simulink model "Neurofeedback_ErrorFunction"  (R2021b)
settings: Solver=VariableStepAuto  StartTime=0.0  StopTime=30  RelTol=1e-3
settings Model: Creator=mariodelossantos  LastModifiedBy=mariodelossantos

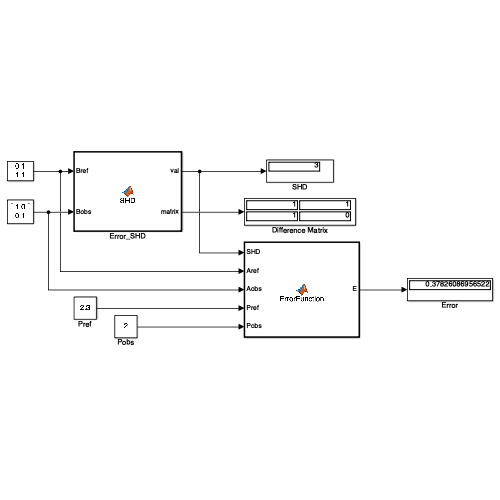
[thumbnail: Simulink's stored preview of the top-level diagram]
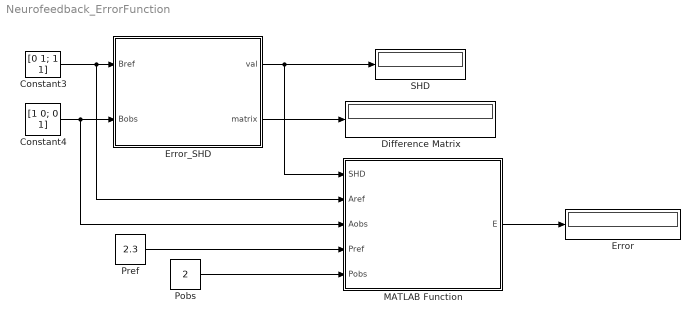
== system Neurofeedback_ErrorFunction ==
  Constant3 : Constant  Value=[0 1; 1 1]
  Constant4 : Constant  Value=[1 0; 0 1]
  Difference Matrix : Display
  Error : Display
  Error_SHD : MATLAB Function  TreatAsAtomicUnit=on
  MATLAB Function : MATLAB Function  TreatAsAtomicUnit=on
  Pobs : Constant  Value=2
  Pref : Constant  Value=2.3
  SHD : Display
  wires:
  Constant4/1 -> MATLAB Function/3(Aobs), Error_SHD/2(Bobs)
  Error_SHD/1(val) -> MATLAB Function/1(SHD), SHD/1
  Error_SHD/2(matrix) -> Difference Matrix/1
  Constant3/1 -> MATLAB Function/2(Aref), Error_SHD/1(Bref)
  MATLAB Function/1(E) -> Error/1
  Pref/1 -> MATLAB Function/4(Pref)
  Pobs/1 -> MATLAB Function/5(Pobs)

== matlab function Neurofeedback_ErrorFunction/Error_SHD ==
  data: Bref input; val output; Bobs input; matrix output
function [val,matrix]=SHD(Bref,Bobs)

val = sum(sum(xor(Bref,Bobs)));
matrix = xor(Bref,Bobs);

== matlab function Neurofeedback_ErrorFunction/MATLAB Function ==
  data: SHD input; Aref input; E output; Aobs input; Pref input; Pobs input
function E  = ErrorFunction(SHD, Aref,Aobs,Pref,Pobs)
    w1 = 0.4; %Use whatever values you like most. Threshold 

    w2 = 1 - w1;

    assert(all(size(Aref) == size(Aobs)));

    assert(size(Aref,1) == size(Aref,2));

    nChannels = size(Aref,1);

    AfullyConnected = ones(nChannels);

    AfullyDisconnected = zeros(nChannels);

    maxDiffSHD = sum(sum(xor(AfullyConnected,AfullyDisconnected))); %SHD

    errA = SHD/maxDiffSHD; %Normalize error in the connectivity

    errP = abs(Pobs-Pref)/abs(Pref);

    
E = w1 * errA + w2 * errP;
